simulink model "EEL_5661_DC_Motor_sJ_PID_velocity_110421"  (R2019a)
settings: Solver=VariableStepAuto  StartTime=0.0  StopTime=0.05  RelTol=1e-3
libraries: simulink x5
settings Model: Creator=rothz  LastModifiedBy=rothz
settings DataIOCC: Refine=5

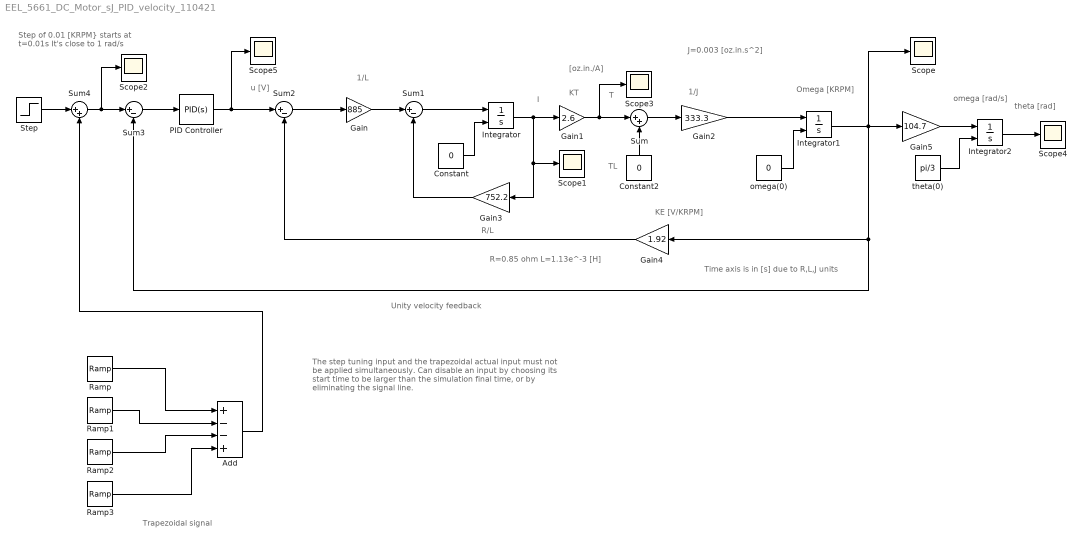
== system EEL_5661_DC_Motor_sJ_PID_velocity_110421 ==
  note: The step tuning input and the trapezoidal actual input must
      | not be applied simultaneously.
      | Can disable an input by choosing its start time to be larger
      | than the simulation final time, or by eliminating the signal line.
  note: Trapezoidal signal
  note: Step of 0.01
      | [KRPM} starts
      | at t=0.01s
      | It's close to 1 rad/s
  note: Unity velocity feedback
  note: omega [rad/s]
  note: theta [rad]
  note: Time axis is in [s] due to R,L,J units
  note: R=0.85 ohm
      | L=1.13e^-3 [H]
  note: [oz.in./A]
  note: J=0.003 [oz.in.s^2]
  note: KE [V/KRPM]
  note: u [V]
  note: 1/L
  note: R/L
  note: I
  note: KT
  note: T
  note: TL
  note: 1/J
  note: Omega [KRPM]
  Add : Sum  Inputs=+--+
  Constant : Constant  Value=0
  Constant2 : Constant  Value=0
  Gain : Gain  Gain=885
  Gain1 : Gain  Gain=2.6
  Gain2 : Gain  Gain=333.3
  Gain3 : Gain  Gain=752.2
  Gain4 : Gain  Gain=1.92
  Gain5 : Gain  Gain=104.7
  Integrator : Integrator  InitialConditionSource=external
  Integrator1 : Integrator  InitialConditionSource=external
  Integrator2 : Integrator  InitialConditionSource=external
  PID Controller : simulink/Continuous/PID Controller  Controller=PID  Form=Parallel  TimeDomain=Continuous-time  SampleTime=-1  IntegratorMethod=Forward Euler  FilterMethod=Forward Euler  ControllerParametersSource=internal  P=1  I=0  D=0  UseFilter=on  N=100  TunerSelectOption=Transfer Function Based (PID Tuner App)  InitialConditionSource=internal  InitialConditionForIntegrator=0  InitialConditionForFilter=0  DifferentiatorICPrevScaledInput=0  ExternalReset=none  TrackingMode=off  Kt=1  LimitOutput=off  UpperSaturationLimit=inf  LowerSaturationLimit=-inf  LinearizeAsGain=on  AntiWindupMode=none  Kb=1  POutMin=[]  POutMax=[]  IOutMin=[]  IOutMax=[]  DOutMin=[]  DOutMax=[]  NOutMin=[]  NOutMax=[]  SumOutMin=[]  SumOutMax=[]  SaturationOutMin=[]  SaturationOutMax=[]  PParamMin=[]  PParamMax=[]  IParamMin=[]  IParamMax=[]  DParamMin=[]  DParamMax=[]  NParamMin=[]  NParamMax=[]  KbParamMin=[]  KbParamMax=[]  KtParamMin=[]  KtParamMax=[]  KbOutMin=[]  KbOutMax=[]  KtOutMin=[]  KtOutMax=[]  IntegratorOutMin=[]  IntegratorOutMax=[]  FilterOutMin=[]  FilterOutMax=[]  SumI1OutMin=[]  SumI1OutMax=[]  SumI2OutMin=[]  SumI2OutMax=[]  SumI3OutMin=[]  SumI3OutMax=[]  SumI4OutMin=[]  SumI4OutMax=[]  SumDOutMin=[]  SumDOutMax=[]  DifferentiatorOutMin=[]  DifferentiatorOutMax=[]  FilterDiffOutCoefMin=[]  FilterDiffOutCoefMax=[]  ReciprocalOutMin=[]  ReciprocalOutMax=[]  SumDenOutMin=[]  SumDenOutMax=[]  SumNumOutMin=[]  SumNumOutMax=[]  DivideOutMin=[]  DivideOutMax=[]  IntegratorContinuousStateAttributes=''  IntegratorStateMustResolveToSignalObject=off  IntegratorRTWStateStorageClass=Auto  FilterContinuousStateAttributes=''  FilterStateMustResolveToSignalObject=off  FilterRTWStateStorageClass=Auto  ParallelPVariant=InternalParameters  IdealPVariant=Disabled  IVariant=InternalParameters  DVariant=InternalParameters  IntegratorVariant=Continuous  SatVariant=Disabled  AWVariant=Passthrough  PCopyVariant=Disabled  TRVariant=Disabled  FdbkBlocksVariant=Forward  IdealPFdbkVariant=Disabled  SatFdbkVariant=Disabled  DerivativeFilterVariant=ContFilter  NVariant=InternalParameters  NCopyVariant=Disabled  FilterICVariant=InternalICsFilter  IntegratorICVariant=InternalICs  ExternalResetVariant=Disabled  TRSumVariant=Passthrough  SumFdbkVariant=Disabled  SumVariant=Sum_PID
  Ramp : simulink/Sources/Ramp  slope=1  start=0.01  InitialOutput=0
  Ramp1 : simulink/Sources/Ramp  slope=1  start=0.02  InitialOutput=0
  Ramp2 : simulink/Sources/Ramp  slope=1  start=0.03  InitialOutput=0
  Ramp3 : simulink/Sources/Ramp  slope=1  start=0.04  InitialOutput=0
  Scope{,1..5} (6 alike) : Scope
  Step : Step  Time=0.01  After=0.01  SampleTime=0
  Sum : Sum  Inputs=|++
  Sum1 : Sum  Inputs=|+-
  Sum2 : Sum  Inputs=|+-
  Sum3 : Sum  Inputs=|+-
  Sum4 : Sum  Inputs=|++
  omega(0) : Constant  Value=0
  theta(0) : Constant  Value=pi/3
  wires:
  Sum2/1 -> Gain/1
  Gain/1 -> Sum1/1
  Sum1/1 -> Integrator/1
  Gain3/1 -> Sum1/2
  Integrator/1 -> Gain1/1, Scope1/1, Gain3/1
  Gain1/1 -> Scope3/1, Sum/1
  Gain2/1 -> Integrator1/1
  Sum/1 -> Gain2/1
  omega(0)/1 -> Integrator1/2
  Constant/1 -> Integrator/2
  Integrator1/1 -> Sum3/2, Gain4/1, Gain5/1, Scope/1
  Constant2/1 -> Sum/2
  Gain4/1 -> Sum2/2
  Sum3/1 -> PID Controller/1
  PID Controller/1 -> Scope5/1, Sum2/1
  Gain5/1 -> Integrator2/1
  Integrator2/1 -> Scope4/1
  theta(0)/1 -> Integrator2/2
  Ramp/1 -> Add/1
  Ramp1/1 -> Add/2
  Ramp2/1 -> Add/3
  Ramp3/1 -> Add/4
  Sum4/1 -> Scope2/1, Sum3/1
  Add/1 -> Sum4/2
  Step/1 -> Sum4/1
